simulink library "lib_two_state_filtered_derivative"  (R2023a)
settings: Solver=VariableStepAuto  StartTime=0.0  StopTime=10.0  RelTol=1e-3
undefined symbols (not defined in the file): bit, lb_parMaxSampTime, parElctAngEstMaxVal, parElctSpdMaxVal, parMedTaskSampTime_u16d6b0, parSpdDrvtCharFreqMaxVal, parSpdDrvtDampCoefMaxVal
libraries: lib_conversion x6, lib_discrete_time_integrator x1
settings Model: Creator=cav2ofo  LastModifiedBy=lenovo
settings OptimizationCC: ReuseModelBlockBuffer=off

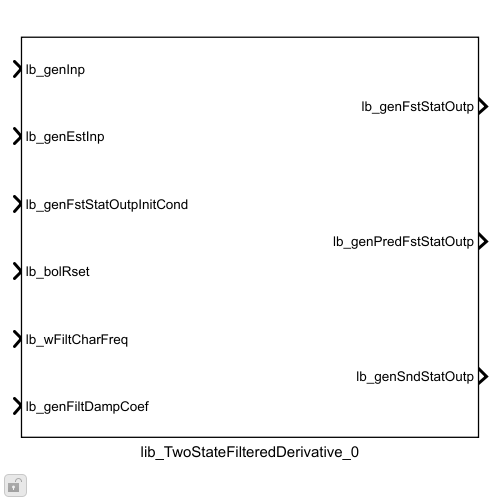
[thumbnail: Simulink's stored preview of the top-level diagram]
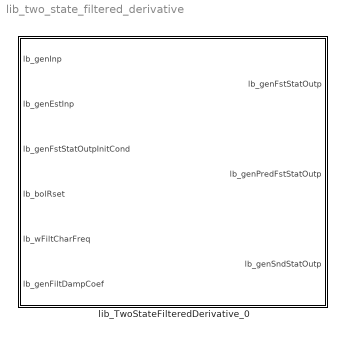
== system lib_two_state_filtered_derivative ==
  lib_TwoStateFilteredDerivative_0 : Subsystem  mask{lb_parSampTime=parMedTaskSampTime_u16d6b0, lb_parMaxSampTime=lb_parMaxSampTime, lb_parMaxCharFreq=parSpdDrvtCharFreqMaxVal, lb_parMaxDampCoef=parSpdDrvtDampCoefMaxVal, lb_parIntgMaxInpVal=lb_parMaxSampTime, lb_parIntgMinInpVal=lb_parMaxSampTime, lb_genFstStatOutpUpLim=parElctSpdMaxVal, lb_genFstStatOutpLowLim=-parElctSpdMaxVal, lb_genInpEstErrMaxVal=parElctAngEstMaxVal, lb_parAngInpMode=on, lb_parAccmDataTypeMode=32-bit, lb_parFstStatOutpDataType=fixdt(1,16,2^-3,0), lb_parSndStatOutpDataType=fixdt(1,16,2^0,0), lb_parIntgScopMode=Integral control, lb_parSatFlag=on}
      mask prompts: lb_parSampTime "Sampling time [s]:"; lb_parMaxSampTime "Maximum sampling time [s]:"; lb_parMaxCharFreq "Maximum characteristic frequency [rad/s]:"; lb_parMaxDampCoef "Maximum damping coefficient:"; lb_parIntgMaxInpVal "Maximum input value [iu]:"; lb_parIntgMinInpVal "Minimum input value [iu]:"; lb_genFstStatOutpUpLim "First state output upper limit [ou]:"; lb_genFstStatOutpLowLim "First state output lower limit [ou]:"; lb_genInpEstErrMaxVal "Maximum input estimation error [iu]:"; lb_parAngInpMode "Angle input mode"; lb_parAccmDataTypeMode "Accumulator data type mode for speed integration:"; lb_parFstStatOutpDataType "First state output data type:"; lb_parSndStatOutpDataType "Second state output data type:"; lb_parIntgScopMode "Integration scope:"; lb_parSatFlag "Output saturation"
      mask init:
      | % % lib_Conversion_4 data type
      | % if strcmp(lb_parInpVrtnDataType.Signedness,'Signed')
      | %     lb_parConv4MaxOutp = double((2^(lb_parInpVrtnDataType.WordLength-1)-1)*...
      | %         lb_parInpVrtnDataType.Slope*lb_parCharFreq);
      | % else
      | %     lb_parConv4MaxOutp = double((2^lb_parInpVrtnDataType.WordLength-1)*...
      | %         lb_parInpVrtnDataType.Slope*lb_parCharFreq);
      | % end
      | % 
      | % % lib_Conversion_5 data type
      | % lb_parConv5MaxOutp = double(lb_parConv4MaxOutp*lb_parDampCoef);
      | % 
      | % % lib_Conversion_6 data type
      | % lb_parConv6MaxOutp = double(lb_parConv5MaxOutp*2);
      | 
      |  
      | temp.inpVrntMaxVal = abs(double(lb_genInpEstErrMaxVal));
      | temp.inpVrntDataType = fi(temp.inpVrntMaxVal);
      | 
      | %% Req. XXX_ - Define data type for input variation
      | lb_parInpVrntDataType = Simulink.NumericType;
      | lb_parInpVrntDataType.DataTypeMode = 'Fixed-point: slope and bias scaling';
      | lb_parInpVrntDataType.Signedness = 'Signed';
      | lb_parInpVrntDataType.WordLength = 16;
      | switch lb_parAngInpMode
      |     case 'on'
      |         lb_parInpVrntDataType.Slope = pi*2^-15;
      |     case 'off'
      |         lb_parInpVrntDataType.Slope = 2^-temp.inpVrntDataType.FractionLength;
      | end
      | 
      | %% Req. XXX_ Define data type for product (u-u_pre)*cf
      | lb_parOper1MaxVal = temp.inpVrntMaxVal*lb_parMaxCharFreq;
      | lb_parOper1DataType = Simulink.NumericType;
      | lb_parOper1DataType.DataTypeMode= 'Fixed-point: unspecified scaling';
      | lb_parOper1DataType.Signedness = 'Signed';
      | lb_parOper1DataType.WordLength = 16;
      | 
      | %% Req. XXX_ Define data type for product (u-u_pre)*cf*dc
      | lb_parOper2MaxVal = temp.inpVrntMaxVal*lb_parMaxCharFreq*lb_parMaxDampCoef;
      | lb_parOper2DataType = Simulink.NumericType;
      | lb_parOper2DataType.DataTypeMode= 'Fixed-point: unspecified scaling';
      | lb_parOper2DataType.Signedness = 'Signed';
      | lb_parOper2DataType.WordLength = 16;
      | 
      | %% Req. XXX_ Define data type for product (u-u_pre)*cf*dc
      | lb_parOper3MaxVal = temp.inpVrntMaxVal*lb_parMaxCharFreq*lb_parMaxDampCoef*2;
      | lb_parOper3DataType = Simulink.NumericType;
      | lb_parOper3DataType.DataTypeMode= 'Fixed-point: unspecified scaling';
      | lb_parOper3DataType.Signedness = 'Signed';
      | lb_parOper3DataType.WordLength = 16;
      | 
      | %% Integrator parameters
      | lb_parIntgMaxInpVal = temp.inpVrntMaxVal*lb_parMaxCharFreq;
      | lb_parIntgMinInpVal = -temp.inpVrntMaxVal*lb_parMaxCharFreq;
      | lb_parMaxSampTime = double(lb_parSampTime);
      | lb_parIntgScopMode = 'Integral control';
      | lb_parSatFlag = true;
      | 
      | %% Manage diagnostics for input variation sum
      | %% Restore any suppressed diagnostics
      | Simulink.restoreDiagnostic(gcb);
      | if strcmp(lb_parAngInpMode,'on')
      |         Simulink.suppressDiagnostic([gcb,'/Add'],...
      |             'SimulinkFixedPoint:util:Overflowoccurred');
      | end
      mask TypeOptions lb_parMaxSampTime: lib_DiscreteTimeIntegrator_1/lb_parMaxSampTime
      mask TypeOptions lb_parMaxCharFreq: lib_DiscreteTimeIntegrator_1/lb_parMaxIntgGain
      mask TypeOptions lb_parIntgMaxInpVal: lib_DiscreteTimeIntegrator_1/lb_parMaxInpVal
      mask TypeOptions lb_parIntgMinInpVal: lib_DiscreteTimeIntegrator_1/lb_parMinInpVal
      mask TypeOptions lb_parAccmDataTypeMode: lib_DiscreteTimeIntegrator_1/lb_parAccmDataTypeMode
      mask TypeOptions lb_parFstStatOutpDataType: lib_DiscreteTimeIntegrator_1/lb_parOutpDataType
      mask TypeOptions lb_parSndStatOutpDataType: lib_Conversion_1/lb_parDataType
      mask TypeOptions lb_parIntgScopMode: lib_DiscreteTimeIntegrator_1/lb_parIntgScopMode
      mask TypeOptions lb_parSatFlag: lib_DiscreteTimeIntegrator_1/lb_parSatFlag
      mask DialogControl DescGroupVar Prompt: VHIT control library
      mask DialogControl DescTextVar Prompt: Two state filtered derivative
      mask DialogControl Container3 Prompt: Data type
      mask DialogControl Container4 Prompt: Operating modes

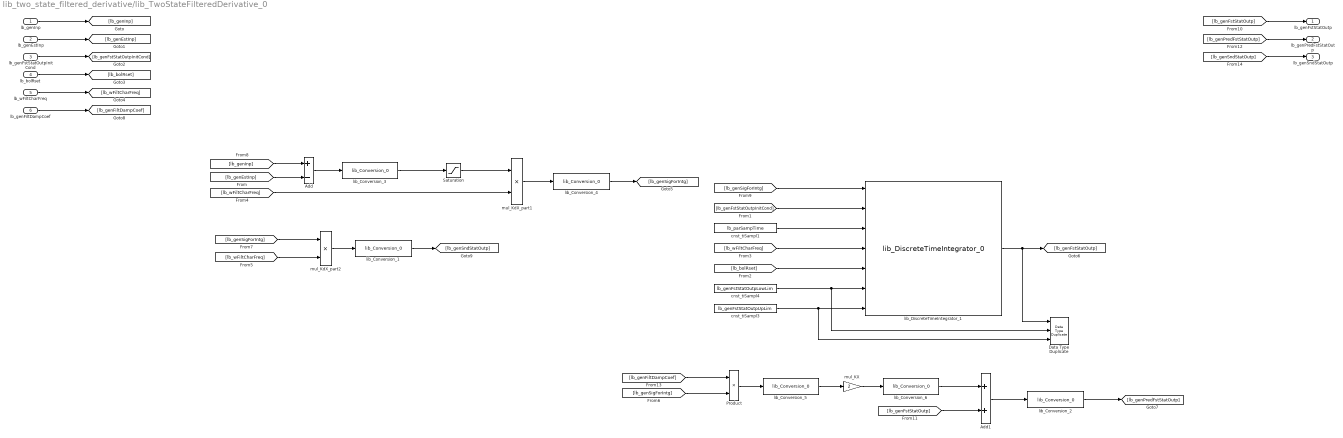
== system lib_two_state_filtered_derivative/lib_TwoStateFilteredDerivative_0 ==
  lb_genInp : Inport  PortDimensions=1
  lb_genEstInp : Inport  Port=2  PortDimensions=1
  lb_genFstStatOutpInitCond : Inport  Port=3  PortDimensions=1
  lb_bolRset : Inport  Port=4  OutDataTypeStr=boolean  PortDimensions=1
  lb_wFiltCharFreq : Inport  Port=5
  lb_genFiltDampCoef : Inport  Port=6
  Add : Sum  Inputs=+-  OutDataTypeStr=Inherit: Inherit via back propagation  RndMeth=Simplest
  Add1 : Sum  OutDataTypeStr=Inherit: Inherit via back propagation  RndMeth=Simplest
  Data Type Duplicate : DataTypeDuplicate  NumInputPorts=3
  Product : Product  OutDataTypeStr=Inherit: Inherit via back propagation  RndMeth=Simplest
  Saturation : Saturate  UpperLimit=lb_genInpEstErrMaxVal  LowerLimit=-lb_genInpEstErrMaxVal  RndMeth=Simplest
  cnst_tiSampl1 : Constant  Value=lb_parSampTime  SampleTime=-1
  cnst_tiSampl3 : Constant  Value=lb_genFstStatOutpUpLim  OutDataTypeStr=Inherit: Inherit via back propagation  SampleTime=-1
  cnst_tiSampl4 : Constant  Value=lb_genFstStatOutpLowLim  OutDataTypeStr=Inherit: Inherit via back propagation  SampleTime=-1
  lib_Conversion_1 : lib_conversion/lib_Conversion_0  lb_parDataType=fixdt(1,16,2^0,0)  lb_parOutpMaxVal=[]  lb_parOutpMinVal=[]  lb_parSatFlag=off
  lib_Conversion_2 : lib_conversion/lib_Conversion_0  lb_parDataType=lb_parFstStatOutpDataType  lb_parOutpMaxVal=[]  lb_parOutpMinVal=[]  lb_parSatFlag=off
  lib_Conversion_3 : lib_conversion/lib_Conversion_0  lb_parDataType=lb_parInpVrntDataType  lb_parOutpMaxVal=[]  lb_parOutpMinVal=[]  lb_parSatFlag=off
  lib_Conversion_4 : lib_conversion/lib_Conversion_0  lb_parDataType=lb_parOper1DataType  lb_parOutpMaxVal=lb_parOper1MaxVal  lb_parOutpMinVal=[]  lb_parSatFlag=off
  lib_Conversion_5 : lib_conversion/lib_Conversion_0  lb_parDataType=lb_parOper2DataType  lb_parOutpMaxVal=lb_parOper2MaxVal  lb_parOutpMinVal=[]  lb_parSatFlag=off
  lib_Conversion_6 : lib_conversion/lib_Conversion_0  lb_parDataType=lb_parOper3DataType  lb_parOutpMaxVal=lb_parOper3MaxVal  lb_parOutpMinVal=[]  lb_parSatFlag=off
  lib_DiscreteTimeIntegrator_1 : lib_discrete_time_integrator/lib_DiscreteTimeIntegrator_0  lb_parMaxInpVal=lb_parIntgMaxInpVal  lb_parMinInpVal=lb_parIntgMinInpVal  lb_parMaxSampTime=lb_parMaxSampTime  lb_parMaxIntgGain=lb_parMaxCharFreq  lb_parAccmDataTypeMode=32-bit  lb_parOutpDataType=fixdt(1,16,2^-3,0)  lb_parIntgScopMode=Integral control  lb_parSatFlag=on
      settings: LibrarySourceBlock=vhit_control_library/lib_DiscreteTimeIntegrator_0
  mul_KX : Gain  Gain=2  OutDataTypeStr=Inherit: Inherit via back propagation  RndMeth=Simplest
  mul_KdX_part1 : Product  OutDataTypeStr=Inherit: Inherit via back propagation  RndMeth=Simplest
  mul_KdX_part2 : Product  OutDataTypeStr=Inherit: Inherit via back propagation  RndMeth=Simplest
  lb_genFstStatOutp : Outport  PortDimensions=1  VectorParamsAs1DForOutWhenUnconnected=off
  lb_genPredFstStatOutp : Outport  Port=2  PortDimensions=1  VectorParamsAs1DForOutWhenUnconnected=off
  lb_genSndStatOutp : Outport  Port=3  PortDimensions=1  VectorParamsAs1DForOutWhenUnconnected=off
  wires:
  Saturation/1 -> mul_KdX_part1/1
  lib_Conversion_5/1 -> mul_KX/1
  [lb_genSigForIntg] -> Product/2
  lb_bolRset/1 -> [lb_bolRset]
  lib_Conversion_3/1 -> Saturation/1
  mul_KdX_part2/1 -> lib_Conversion_1/1
  [lb_wFiltCharFreq] -> lib_DiscreteTimeIntegrator_1/4
  lb_genFstStatOutpInitCond/1 -> [lb_genFstStatOutpInitCond]
  mul_KdX_part1/1 -> lib_Conversion_4/1
  mul_KX/1 -> lib_Conversion_6/1
  Add/1 -> lib_Conversion_3/1
  lib_DiscreteTimeIntegrator_1/1 -> [lb_genFstStatOutp], Data Type Duplicate/1
  cnst_tiSampl1/1 -> lib_DiscreteTimeIntegrator_1/3
  Product/1 -> lib_Conversion_5/1
  cnst_tiSampl4/1 -> lib_DiscreteTimeIntegrator_1/6, Data Type Duplicate/2
  cnst_tiSampl3/1 -> lib_DiscreteTimeIntegrator_1/7, Data Type Duplicate/3
  lb_genInp/1 -> [lb_genInp]
  lb_genEstInp/1 -> [lb_genEstInp]
  [lb_genInp] -> Add/1
  [lb_genEstInp] -> Add/2
  [lb_genFstStatOutpInitCond] -> lib_DiscreteTimeIntegrator_1/2
  [lb_bolRset] -> lib_DiscreteTimeIntegrator_1/5
  lb_wFiltCharFreq/1 -> [lb_wFiltCharFreq]
  [lb_wFiltCharFreq] -> mul_KdX_part1/2
  [lb_wFiltCharFreq] -> mul_KdX_part2/2
  lib_Conversion_4/1 -> [lb_genSigForIntg]
  [lb_genSigForIntg] -> mul_KdX_part2/1
  [lb_genSigForIntg] -> lib_DiscreteTimeIntegrator_1/1
  [lb_genFstStatOutp] -> lb_genFstStatOutp/1
  lib_Conversion_6/1 -> Add1/1
  [lb_genFstStatOutp] -> Add1/2
  Add1/1 -> lib_Conversion_2/1
  [lb_genPredFstStatOutp] -> lb_genPredFstStatOutp/1
  lib_Conversion_2/1 -> [lb_genPredFstStatOutp]
  lb_genFiltDampCoef/1 -> [lb_genFiltDampCoef]
  [lb_genFiltDampCoef] -> Product/1
  [lb_genSndStatOutp] -> lb_genSndStatOutp/1
  lib_Conversion_1/1 -> [lb_genSndStatOutp]
